simulink model "eval_nets_2019a"  (R2019a)
settings: Solver=FixedStepAuto  StartTime=0.0  StopTime=10.0  FixedStep=1/400  RelTol=1e-3
settings Model: Creator=brandlju  LastModifiedBy=brandlju
settings OptimizationCC: LocalBlockOutputs=off
settings RTWCC: SystemTargetFile=TwinCAT.tlc  GenCodeOnly=on  MakeCommand=make_tct  TemplateMakefile=tct_msbuild.tmf  Description=TwinCAT Target  GenerateReport=on  TargetLang=C++
settings STFCustomTargetCC: TargetLangStandard=C++03 (ISO)  CompOptLevelCompliant=on  MATLABClassNameForMDSCustomization=Simulink.SoftwareTarget.TargetSpecificTriggerConfigurationBase  SystemTargetFile=TwinCAT.tlc

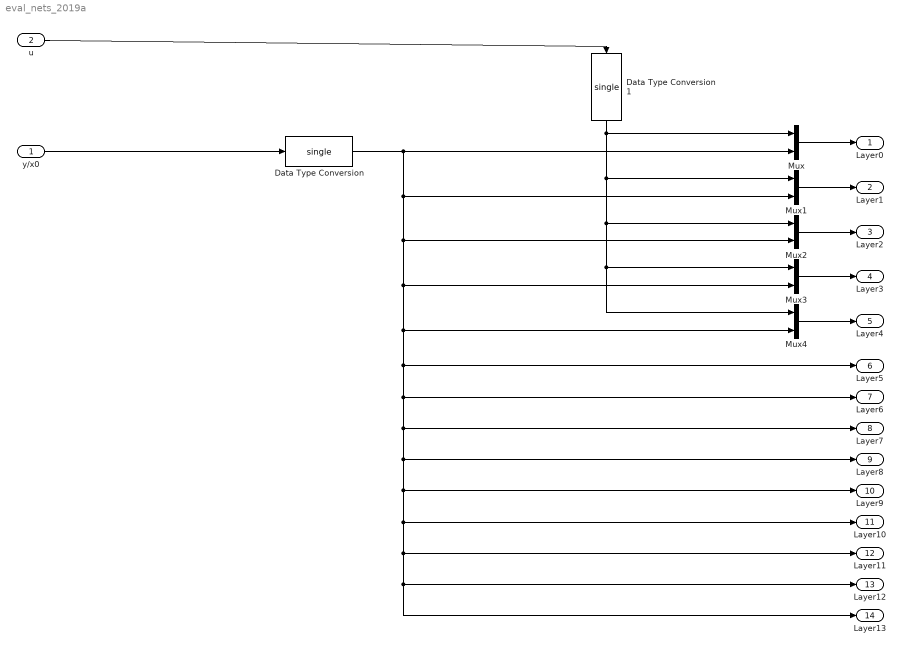
== system eval_nets_2019a ==
  y/x0 : Inport  OutDataTypeStr=double  PortDimensions=1
  u : Inport  Port=2  OutDataTypeStr=double
  Data Type Conversion : DataTypeConversion  OutDataTypeStr=single
  Data Type Conversion1 : DataTypeConversion  OutDataTypeStr=single
  Mux{,1..4} (5 alike) : Mux  Inputs=2
  Layer0 : Outport  OutDataTypeStr=single  PortDimensions=2  VectorParamsAs1DForOutWhenUnconnected=on
  Layer1 : Outport  Port=2  OutDataTypeStr=single  PortDimensions=2  VectorParamsAs1DForOutWhenUnconnected=on
  Layer2 : Outport  Port=3  OutDataTypeStr=single  PortDimensions=2  VectorParamsAs1DForOutWhenUnconnected=on
  Layer3 : Outport  Port=4  OutDataTypeStr=single  PortDimensions=2  VectorParamsAs1DForOutWhenUnconnected=on
  Layer4 : Outport  Port=5  OutDataTypeStr=single  PortDimensions=2  VectorParamsAs1DForOutWhenUnconnected=on
  Layer5 : Outport  Port=6  OutDataTypeStr=single  PortDimensions=1  VectorParamsAs1DForOutWhenUnconnected=on
  Layer6 : Outport  Port=7  OutDataTypeStr=single  PortDimensions=1  VectorParamsAs1DForOutWhenUnconnected=on
  Layer7 : Outport  Port=8  OutDataTypeStr=single  PortDimensions=1  VectorParamsAs1DForOutWhenUnconnected=on
  Layer8 : Outport  Port=9  OutDataTypeStr=single  PortDimensions=1  VectorParamsAs1DForOutWhenUnconnected=on
  Layer9 : Outport  Port=10  OutDataTypeStr=single  PortDimensions=1  VectorParamsAs1DForOutWhenUnconnected=on
  Layer10 : Outport  Port=11  OutDataTypeStr=single  PortDimensions=1  VectorParamsAs1DForOutWhenUnconnected=on
  Layer11 : Outport  Port=12  OutDataTypeStr=single  PortDimensions=1  VectorParamsAs1DForOutWhenUnconnected=on
  Layer12 : Outport  Port=13  OutDataTypeStr=single  PortDimensions=1  VectorParamsAs1DForOutWhenUnconnected=on
  Layer13 : Outport  Port=14  OutDataTypeStr=single  PortDimensions=1  VectorParamsAs1DForOutWhenUnconnected=on
  wires:
  y/x0/1 -> Data Type Conversion/1
  Mux1/1 -> Layer1/1
  Data Type Conversion1/1 -> Mux4/1, Mux3/1, Mux2/1, Mux1/1, Mux/1
  Mux4/1 -> Layer4/1
  Mux/1 -> Layer0/1
  Data Type Conversion/1 -> Layer5/1, Layer6/1, Layer7/1, Layer8/1, Layer9/1, Layer10/1, Layer11/1, Layer12/1, Layer13/1, Mux4/2, Mux3/2, Mux2/2, Mux1/2, Mux/2
  Mux2/1 -> Layer2/1
  Mux3/1 -> Layer3/1
  u/1 -> Data Type Conversion1/1
